simulink model "hw2pendulumNL"  (R2013b)
settings: Solver=ode45  StartTime=0.0  StopTime=100  RelTol=1e-3
settings Model: Creator=czhang  LastModifiedBy=czhang

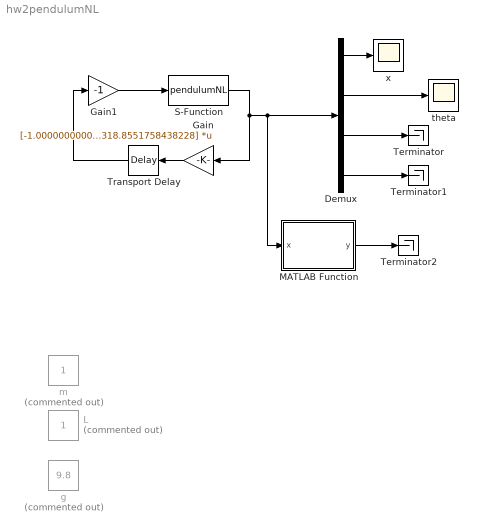
== system hw2pendulumNL ==
  Demux : Demux
  Gain : Gain  Gain="[-1.0000000000022 -325.6026451744055 -6.7416258738856  -318.8551758438228]"  Multiplication=Matrix(K*u)
  Gain1 : Gain  Gain=-1
  L : Constant  Commented=on
  MATLAB Function : MATLAB Function  TreatAsAtomicUnit=on
  S-Function : S-Function  FunctionName=pendulumNL  EnableBusSupport=off
  Terminator : Terminator
  Terminator1 : Terminator
  Terminator2 : Terminator
  Transport Delay : TransportDelay  DelayTime=.28
  g : Constant  Commented=on  Value=9.8
  m : Constant  Commented=on
  theta : Scope
  x : Scope
  wires:
  Demux/4 -> Terminator1/1
  Demux/3 -> Terminator/1
  Demux/2 -> theta/1
  Demux/1 -> x/1
  Gain/1 -> Transport Delay/1
  Transport Delay/1 -> Gain1/1
  S-Function/1 -> MATLAB Function/1(x), Demux/1, Gain/1
  Gain1/1 -> S-Function/1
  MATLAB Function/1(y) -> Terminator2/1

== matlab function hw2pendulumNL/MATLAB Function ==
  data: x input size=4; y output
function y = fcn(x)
y = x;
figure(1); hold off; %clf reset
% setupGCF();

drawnow
xMin = -1.5; xMax = 1.5; cartWidth = .25; cartHeight = .1;
cla reset;axis([xMin,xMax,-.5,1.5]); axis('off')
set(1,'Color','k');

% Draw bottom
% line([xMin,xMax],[0,0],'EraseMode','xor','LineStyle','-','Color','w');
line([xMin,xMax],[-cartHeight,-cartHeight],...
    'EraseMode','xor','LineStyle','-','Color','w');

% Draw cart
cartXLeft = x(1)-cartWidth/2;
cartXRight = x(1)+cartWidth/2;
line([cartXLeft,cartXRight],[-cartHeight,-cartHeight]/2,...
    'EraseMode','xor','LineStyle','-','Color','r','LineWidth',15);

% Draw pendulum
pendXBot = x(1);
pendXTop = x(1)+L*sin(x(2));
pendYBot = 0;
pendYTop = L*cos(x(2));
line([pendXBot,pendXTop],[pendYBot,pendYTop],...
    'EraseMode','xor','LineStyle','-','Color','b','LineWidth',5);
